simulink model "SVPWM_Three_Phase_Two_Level_Inverter"  (R2022a)
settings: Solver=VariableStepAuto  StartTime=0.0  StopTime=1  FixedStep=1e-5  RelTol=1e-3
libraries: spsIGBTLib x6, spsSeriesRLCBranchLib x3, spsPLLLib x1, simulink x1, spsDCVoltageSourceLib x1, spsGroundLib x1, spsThreePhaseVIMeasurementLib x1, spspowerguiLib x1
settings Model: Creator=nikos  LastModifiedBy=nikos

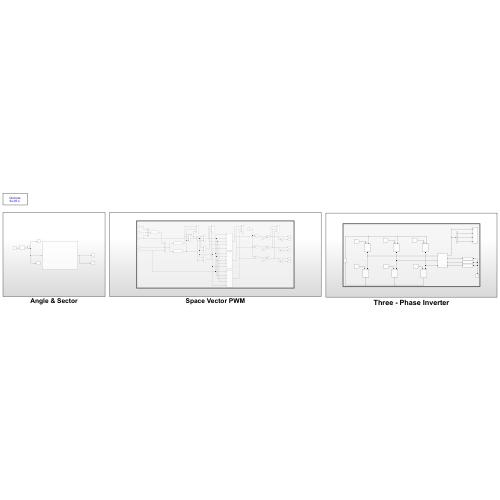
[thumbnail: Simulink's stored preview of the top-level diagram]
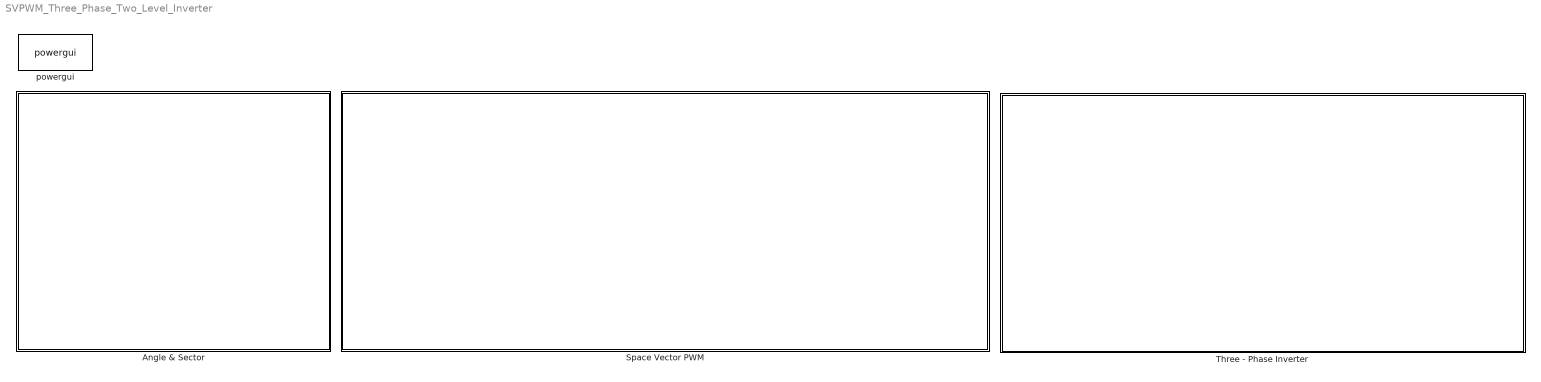
== system SVPWM_Three_Phase_Two_Level_Inverter ==
  Angle & Sector : Subsystem
  Space Vector PWM : Subsystem
  Three - Phase Inverter : Subsystem
  powergui : spspowerguiLib/powergui  Priority=1  SimulationMode=Discrete  SampleTime=50e-6  frequency=60  Iterations=50  frequencyindice=0  Pbase=100e6  ErrMax=1e-4  UnitsV=kV  UnitsW=MW  buscounter=0  FunctionMessages=off  echomessages=off  EnableUseOfTLC=off  CurrentSourceSwitches=off  DisableSnubberDevices=off  DisableRonSwitches=off  DisableVfSwitches=off  DisplayEquations=off  AutomaticDiscreteSolvers=off  SolverType=Tustin/Backward Euler (TBE)  Interpol=off  ExternalGateDelay=off  methode=off  Ts=100  x0status=blocks  SPID=on  SwTol=0  HookPort=off  NonlinearTolerance=1e-4  nMaxIteration=100  ContinueOnMaxIteration=off  RestoreLinks=warning  ResistiveCurrentMeasurement=off  Frange=[0:2:500]  Ylog=off  Xlog=on  ShowGrid=off  save=off  variable=ZData  structure=0  ZoomFFT=off  StartTime=0.0  cycles=1  DisplayStyle=1  fundamental=60  FreqAxis=off  MaxFrequency=1000  frequencyindicesteady=1  RmsSteady=1  display=off

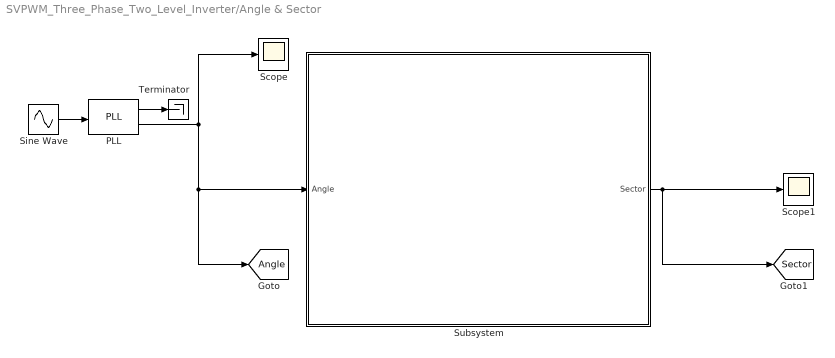
== system SVPWM_Three_Phase_Two_Level_Inverter/Angle & Sector ==
  PLL : spsPLLLib/PLL  Fmin=45  Par_Init=[0, 60]  ParK=[180, 3200, 1]  TcD=1e-4  MaxRateChangeFreq=12  FilterCutOffFreq=25  Ts=0  AGC=on
      settings: SourceProductBaseCode=PS
  Scope : Scope
  Scope1 : Scope
  Sine Wave : Sin  Frequency=2*pi*50  SampleTime=0
  Subsystem : Subsystem
  Terminator : Terminator
  tag scope: Angle=global, Sector=global
  wires:
  PLL/2 -> [Angle], Subsystem/1(Angle), Scope/1
  PLL/1 -> Terminator/1
  Sine Wave/1 -> PLL/1
  Subsystem/1(Sector) -> [Sector], Scope1/1

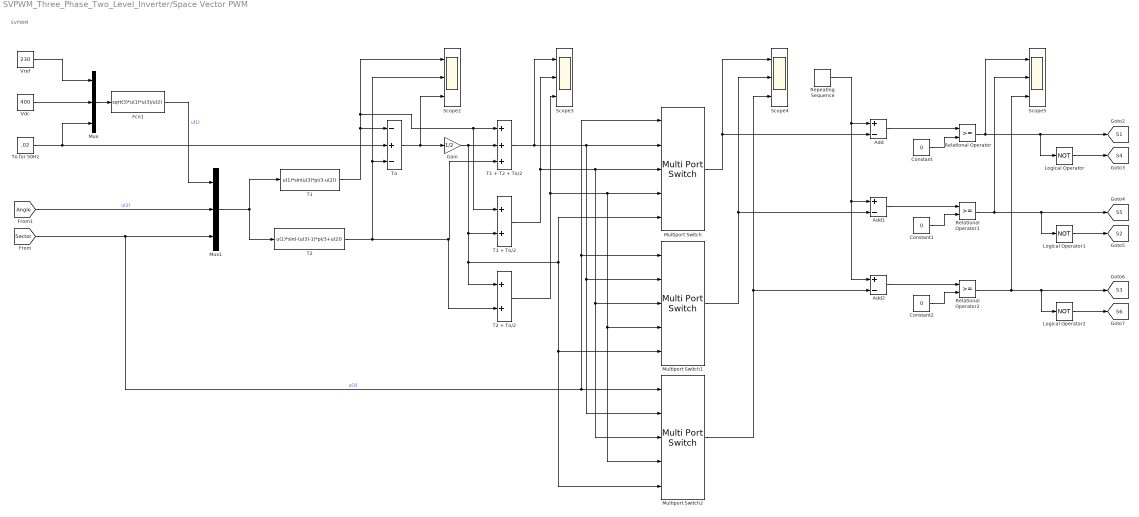
== system SVPWM_Three_Phase_Two_Level_Inverter/Space Vector PWM ==
  note: SVPWM
  Add : Sum  Inputs=+-
  Add1 : Sum  Inputs=+-
  Add2 : Sum  Inputs=+-
  Constant : Constant  Value=0
  Constant1 : Constant  Value=0
  Constant2 : Constant  Value=0
  Fcn1 : Fcn  Expr=sqrt(3)*u(1)*u(3)/u(2)
  Gain : Gain  Gain=1/2
  Logical Operator : Logic  Operator=NOT  AllPortsSameDT=off  OutDataTypeStr=boolean
  Logical Operator1 : Logic  Operator=NOT  AllPortsSameDT=off  OutDataTypeStr=boolean
  Logical Operator2 : Logic  Operator=NOT  AllPortsSameDT=off  OutDataTypeStr=boolean
  Multiport Switch : MultiPortSwitch  DataPortOrder=Specify indices  DataPortIndices={[1,6],2,5,[3,4]}  SaturateOnIntegerOverflow=off  InputSameDT=off
  Multiport Switch1 : MultiPortSwitch  DataPortOrder=Specify indices  DataPortIndices={[2,3],4,1,[5,6]}  SaturateOnIntegerOverflow=off  InputSameDT=off
  Multiport Switch2 : MultiPortSwitch  DataPortOrder=Specify indices  DataPortIndices={[4,5],6,3,[1,2]}  SaturateOnIntegerOverflow=off  InputSameDT=off
  Mux : Mux  Inputs=3
  Mux1 : Mux  Inputs=3
  Relational Operator : RelationalOperator  OutDataTypeStr=boolean  RndMeth=Simplest  InputSameDT=off
  Relational Operator1 : RelationalOperator  OutDataTypeStr=boolean  RndMeth=Simplest  InputSameDT=off
  Relational Operator2 : RelationalOperator  OutDataTypeStr=boolean  RndMeth=Simplest  InputSameDT=off
  Repeating Sequence : simulink/Sources/Repeating Sequence  rep_seq_t=[0 .001]  rep_seq_y=[0 .02]
  Scope{2..5} (4 alike) : Scope  NumInputPorts=3
  T1 : Fcn  Expr=u(1)*sin(u(3)*pi/3-u(2))
  T1 + T2 + To/2 : Sum  Inputs=+++
  T1 + To/2 : Sum
  T2 : Fcn  Expr=u(1)*sin(-(u(3)-1)*pi/3+u(2))
  T2 + To/2 : Sum
  To : Sum  Inputs=-+-
  To for 50Hz : Constant  Value=.02
  Vdc : Constant  Value=400
  Vref : Constant  Value=230
  tag scope: S1=global, S2=global, S3=global, S4=global, S5=global, S6=global
  wires:
  Logical Operator1/1 -> [S2]
  Vref/1 -> Mux/1
  Multiport Switch1/1 -> Add1/2, Scope4/2
  To for 50Hz/1 -> To/2, Mux/3
  T2 + To/2/1 -> Multiport Switch2/4, Multiport Switch1/4, Multiport Switch/4, Scope3/3
  Relational Operator1/1 -> Logical Operator1/1, [S5], Scope5/2
  Vdc/1 -> Mux/2
  T1 + To/2/1 -> Multiport Switch2/3, Multiport Switch1/3, Multiport Switch/3, Scope3/2
  T2/1 -> Scope2/2, To/3, T2 + To/2/2, T1 + T2 + To/2/3
  Add2/1 -> Relational Operator2/1
  Gain/1 -> T1 + To/2/2, T2 + To/2/1, Multiport Switch2/5, Multiport Switch1/5, Multiport Switch/5, T1 + T2 + To/2/2
  Relational Operator2/1 -> Logical Operator2/1, [S3], Scope5/3
  T1 + T2 + To/2/1 -> Multiport Switch2/2, Multiport Switch1/2, Multiport Switch/2, Scope3/1
  [Sector] -> Multiport Switch2/1, Multiport Switch/1, Multiport Switch1/1, Mux1/3  "u(3)"
  Add1/1 -> Relational Operator1/1
  Logical Operator/1 -> [S4]
  Multiport Switch/1 -> Add/2, Scope4/1
  Multiport Switch2/1 -> Scope4/3, Add2/2
  Fcn1/1 -> Mux1/1  "u(1)"
  Add/1 -> Relational Operator/1
  Mux/1 -> Fcn1/1
  Logical Operator2/1 -> [S6]
  T1/1 -> To/1, T1 + To/2/1, T1 + T2 + To/2/1, Scope2/1
  Relational Operator/1 -> Logical Operator/1, [S1], Scope5/1
  [Angle] -> Mux1/2  "u(2)"
  Mux1/1 -> T2/1, T1/1
  Constant2/1 -> Relational Operator2/2
  To/1 -> Scope2/3, Gain/1
  Constant1/1 -> Relational Operator1/2
  Constant/1 -> Relational Operator/2
  Repeating Sequence/1 -> Add2/1, Add1/1, Add/1

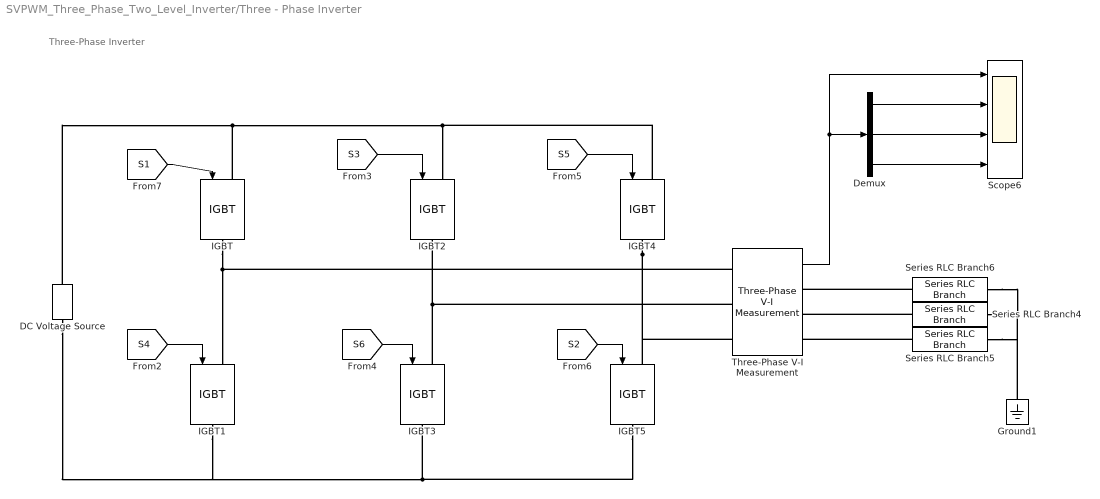
== system SVPWM_Three_Phase_Two_Level_Inverter/Three - Phase Inverter ==
  note: Three-Phase Inverter
  DC Voltage Source : spsDCVoltageSourceLib/DC Voltage Source  Amplitude=400  Measurements=None
  Demux : Demux  Outputs=3
  Ground1 : spsGroundLib/Ground  LConnTagsString=a
  IGBT{,1..5} (6 alike) : spsIGBTLib/IGBT  Ron=0.001  Lon=0  Vf=1  Tf=1e-6  Tt=2e-6  IC=0  Rs=1e5  Cs=inf  Measurements=off
  Scope6 : Scope  NumInputPorts=4
  Series RLC Branch4 : spsSeriesRLCBranchLib/Series RLC Branch  LConnTagsString=__new0  RConnTagsString=__new0  BranchType=R  Resistance=100  Inductance=1e-3  SetiL0=off  InitialCurrent=0  Capacitance=1e-6  Setx0=off  InitialVoltage=0  Measurements=None
  Series RLC Branch5 : spsSeriesRLCBranchLib/Series RLC Branch  LConnTagsString=__new0  RConnTagsString=__new0  BranchType=R  Resistance=100  Inductance=1e-3  SetiL0=off  InitialCurrent=0  Capacitance=1e-6  Setx0=off  InitialVoltage=0  Measurements=None
  Series RLC Branch6 : spsSeriesRLCBranchLib/Series RLC Branch  LConnTagsString=__new0  RConnTagsString=__new0  BranchType=R  Resistance=100  Inductance=1e-3  SetiL0=off  InitialCurrent=0  Capacitance=1e-6  Setx0=off  InitialVoltage=0  Measurements=None
  Three-Phase V-I Measurement : spsThreePhaseVIMeasurementLib/Three-Phase V-I Measurement  VoltageMeasurement=phase-to-ground  SetLabelV=off  LabelV=Vabc  Vpu=off  VpuLL=off  CurrentMeasurement=no  SetLabelI=off  LabelI=Iabc  Ipu=off  Pbase=100e6  Vbase=500e3  OutputType=Complex  PhasorSimulation=off  PSBequivalent=0
  wires:
  Demux/1 -> Scope6/2
  Three-Phase V-I Measurement/1 -> Demux/1, Scope6/1
  Demux/3 -> Scope6/4
  [S5] -> IGBT4/1
  [S4] -> IGBT1/1
  [S1] -> IGBT/1
  [S3] -> IGBT2/1
  [S2] -> IGBT5/1
  [S6] -> IGBT3/1
  Demux/2 -> Scope6/3
  connections:
  Three-Phase V-I Measurement/LConn2 -- IGBT2/RConn1 -- IGBT3/LConn1
  IGBT5/RConn1 -- IGBT3/RConn1 -- DC Voltage Source/LConn1 -- IGBT1/RConn1
  IGBT4/RConn1 -- Three-Phase V-I Measurement/LConn3 -- IGBT5/LConn1
  Series RLC Branch5/RConn1 -- Three-Phase V-I Measurement/RConn3
  Three-Phase V-I Measurement/LConn1 -- IGBT1/LConn1 -- IGBT/RConn1
  IGBT/LConn1 -- DC Voltage Source/RConn1 -- IGBT2/LConn1 -- IGBT4/LConn1
  Series RLC Branch4/RConn1 -- Three-Phase V-I Measurement/RConn2
  Series RLC Branch6/LConn1 -- Series RLC Branch4/LConn1 -- Ground1/LConn1 -- Series RLC Branch5/LConn1
  Series RLC Branch6/RConn1 -- Three-Phase V-I Measurement/RConn1

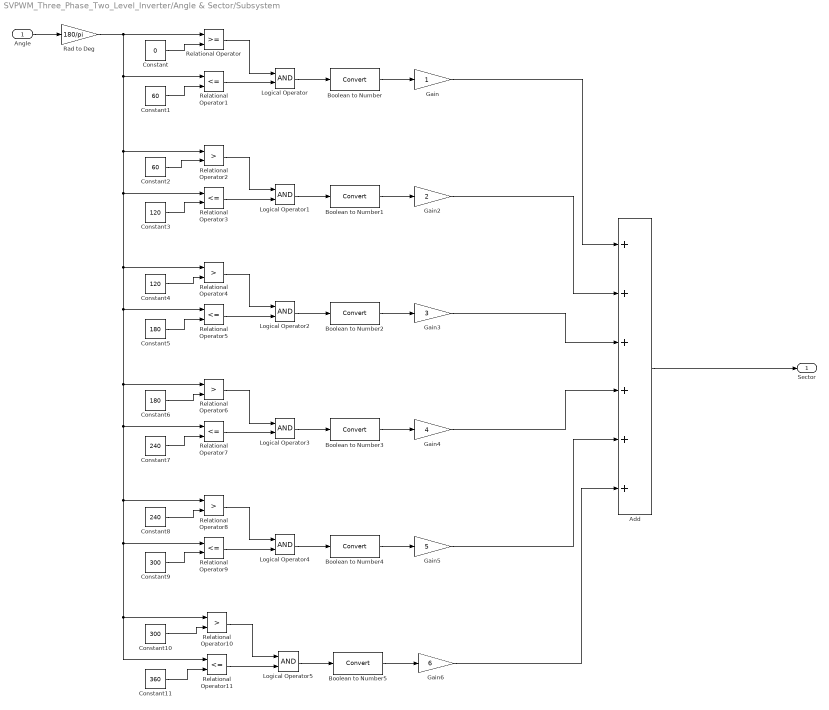
== system SVPWM_Three_Phase_Two_Level_Inverter/Angle & Sector/Subsystem ==
  Angle : Inport
  Add : Sum  Inputs=++++++
  Boolean to Number{,1..5} (6 alike) : DataTypeConversion  SaturateOnIntegerOverflow=off  RndMeth=Floor
  Constant : Constant  Value=0
  Constant1 : Constant  Value=60
  Constant10 : Constant  Value=300
  Constant11 : Constant  Value=360
  Constant2 : Constant  Value=60
  Constant3 : Constant  Value=120
  Constant4 : Constant  Value=120
  Constant5 : Constant  Value=180
  Constant6 : Constant  Value=180
  Constant7 : Constant  Value=240
  Constant8 : Constant  Value=240
  Constant9 : Constant  Value=300
  Gain : Gain
  Gain2 : Gain  Gain=2
  Gain3 : Gain  Gain=3
  Gain4 : Gain  Gain=4
  Gain5 : Gain  Gain=5
  Gain6 : Gain  Gain=6
  Logical Operator{,1..5} (6 alike) : Logic  AllPortsSameDT=off  OutDataTypeStr=boolean
  Rad to Deg : Gain  Gain=180/pi
  Relational Operator : RelationalOperator  OutDataTypeStr=boolean  RndMeth=Simplest  InputSameDT=off
  Relational Operator{1,3,5,7,9,11} (6 alike) : RelationalOperator  Operator=<=  OutDataTypeStr=boolean  RndMeth=Simplest  InputSameDT=off
  Relational Operator{2,4,6,8,10} (5 alike) : RelationalOperator  Operator=>  OutDataTypeStr=boolean  RndMeth=Simplest  InputSameDT=off
  Sector : Outport
  wires:
  Angle/1 -> Rad to Deg/1
  Constant/1 -> Relational Operator/2
  Constant1/1 -> Relational Operator1/2
  Relational Operator/1 -> Logical Operator/1
  Relational Operator1/1 -> Logical Operator/2
  Logical Operator/1 -> Boolean to Number/1
  Boolean to Number/1 -> Gain/1
  Boolean to Number1/1 -> Gain2/1
  Logical Operator1/1 -> Boolean to Number1/1
  Relational Operator3/1 -> Logical Operator1/2
  Relational Operator2/1 -> Logical Operator1/1
  Constant3/1 -> Relational Operator3/2
  Constant2/1 -> Relational Operator2/2
  Constant4/1 -> Relational Operator4/2
  Constant5/1 -> Relational Operator5/2
  Relational Operator4/1 -> Logical Operator2/1
  Relational Operator5/1 -> Logical Operator2/2
  Logical Operator2/1 -> Boolean to Number2/1
  Boolean to Number2/1 -> Gain3/1
  Boolean to Number3/1 -> Gain4/1
  Logical Operator3/1 -> Boolean to Number3/1
  Relational Operator7/1 -> Logical Operator3/2
  Relational Operator6/1 -> Logical Operator3/1
  Constant7/1 -> Relational Operator7/2
  Constant6/1 -> Relational Operator6/2
  Constant8/1 -> Relational Operator8/2
  Constant9/1 -> Relational Operator9/2
  Relational Operator8/1 -> Logical Operator4/1
  Relational Operator9/1 -> Logical Operator4/2
  Logical Operator4/1 -> Boolean to Number4/1
  Boolean to Number4/1 -> Gain5/1
  Boolean to Number5/1 -> Gain6/1
  Logical Operator5/1 -> Boolean to Number5/1
  Relational Operator11/1 -> Logical Operator5/2
  Relational Operator10/1 -> Logical Operator5/1
  Constant11/1 -> Relational Operator11/2
  Constant10/1 -> Relational Operator10/2
  Rad to Deg/1 -> Relational Operator/1, Relational Operator10/1, Relational Operator11/1, Relational Operator9/1, Relational Operator8/1, Relational Operator7/1, Relational Operator6/1, Relational Operator5/1, Relational Operator4/1, Relational Operator3/1, Relational Operator2/1, Relational Operator1/1
  Gain/1 -> Add/1
  Gain2/1 -> Add/2
  Gain3/1 -> Add/3
  Gain4/1 -> Add/4
  Gain5/1 -> Add/5
  Gain6/1 -> Add/6
  Add/1 -> Sector/1
